simulink model "AccelCtrl_ACC_2018b"  (R2018b)
settings: Solver=FixedStepAuto  StartTime=0.0  StopTime=inf  FixedStep=0.001  RelTol=1e-3  EnableMultiTasking=on
libraries: CarMaker4SL x42, simulink x2
(part 2 of 3)

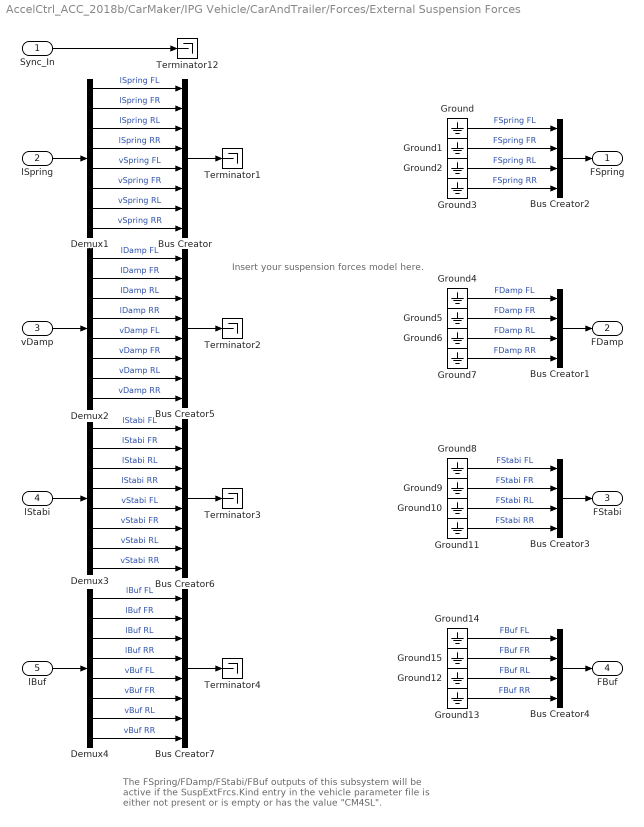
== system AccelCtrl_ACC_2018b/CarMaker/IPG Vehicle/CarAndTrailer/Forces/External Suspension Forces ==
  note: The FSpring/FDamp/FStabi/FBuf outputs of this subsystem will be
      | active if the SuspExtFrcs.Kind entry in the vehicle parameter file
      | is either not present or is empty or has the value "CM4SL".
  note: Insert your suspension forces model here.
  Sync_In : Inport
  lSpring : Inport  Port=2
  vDamp : Inport  Port=3
  lStabi : Inport  Port=4
  lBuf : Inport  Port=5
  Bus Creator{,5..7} (4 alike) : BusCreator  Inputs=8
  Bus Creator{1..4} (4 alike) : BusCreator  Inputs=4
  Demux{1..4} (4 alike) : Demux  Outputs=8
  Ground{,1..15} (16 alike) : Ground
  Terminator{1..4,12} (5 alike) : Terminator
  FSpring : Outport
  FDamp : Outport  Port=2
  FStabi : Outport  Port=3
  FBuf : Outport  Port=4
  wires:
  Bus Creator7/1 -> Terminator4/1
  Bus Creator6/1 -> Terminator3/1
  Bus Creator5/1 -> Terminator2/1
  Bus Creator/1 -> Terminator1/1
  Demux4/8 -> Bus Creator7/8  "vBuf RR"
  Demux4/7 -> Bus Creator7/7  "vBuf RL"
  Demux4/6 -> Bus Creator7/6  "vBuf FR"
  Demux4/5 -> Bus Creator7/5  "vBuf FL"
  Demux3/8 -> Bus Creator6/8  "vStabi RR"
  Demux3/7 -> Bus Creator6/7  "vStabi RL"
  Demux3/6 -> Bus Creator6/6  "vStabi FR"
  Demux3/5 -> Bus Creator6/5  "vStabi FL"
  Demux2/8 -> Bus Creator5/8  "vDamp RR"
  Demux2/7 -> Bus Creator5/7  "vDamp RL"
  Demux2/6 -> Bus Creator5/6  "vDamp FR"
  Demux2/5 -> Bus Creator5/5  "vDamp FL"
  Demux1/8 -> Bus Creator/8  "vSpring RR"
  Demux1/7 -> Bus Creator/7  "vSpring RL"
  Demux1/6 -> Bus Creator/6  "vSpring FR"
  Demux1/5 -> Bus Creator/5  "vSpring FL"
  Demux2/4 -> Bus Creator5/4  "lDamp RR"
  Demux2/3 -> Bus Creator5/3  "lDamp RL"
  Demux2/2 -> Bus Creator5/2  "lDamp FR"
  Demux2/1 -> Bus Creator5/1  "lDamp FL"
  Demux1/4 -> Bus Creator/4  "lSpring RR"
  Demux1/3 -> Bus Creator/3  "lSpring RL"
  Demux1/2 -> Bus Creator/2  "lSpring FR"
  Demux1/1 -> Bus Creator/1  "lSpring FL"
  Demux3/4 -> Bus Creator6/4  "lStabi RR"
  Demux3/3 -> Bus Creator6/3  "lStabi RL"
  Demux3/2 -> Bus Creator6/2  "lStabi FR"
  Demux3/1 -> Bus Creator6/1  "lStabi FL"
  lStabi/1 -> Demux3/1
  vDamp/1 -> Demux2/1
  lSpring/1 -> Demux1/1
  Demux4/4 -> Bus Creator7/4  "lBuf RR"
  Demux4/3 -> Bus Creator7/3  "lBuf RL"
  Demux4/2 -> Bus Creator7/2  "lBuf FR"
  Demux4/1 -> Bus Creator7/1  "lBuf FL"
  lBuf/1 -> Demux4/1
  Ground14/1 -> Bus Creator4/1  "FBuf FL"
  Ground15/1 -> Bus Creator4/2  "FBuf FR"
  Ground12/1 -> Bus Creator4/3  "FBuf RL"
  Ground13/1 -> Bus Creator4/4  "FBuf RR"
  Bus Creator4/1 -> FBuf/1
  Sync_In/1 -> Terminator12/1
  Bus Creator2/1 -> FSpring/1
  Ground/1 -> Bus Creator2/1  "FSpring FL"
  Ground1/1 -> Bus Creator2/2  "FSpring FR"
  Ground2/1 -> Bus Creator2/3  "FSpring RL"
  Ground3/1 -> Bus Creator2/4  "FSpring RR"
  Ground4/1 -> Bus Creator1/1  "FDamp FL"
  Ground5/1 -> Bus Creator1/2  "FDamp FR"
  Ground6/1 -> Bus Creator1/3  "FDamp RL"
  Ground7/1 -> Bus Creator1/4  "FDamp RR"
  Bus Creator1/1 -> FDamp/1
  Ground8/1 -> Bus Creator3/1  "FStabi FL"
  Ground9/1 -> Bus Creator3/2  "FStabi FR"
  Ground10/1 -> Bus Creator3/3  "FStabi RL"
  Ground11/1 -> Bus Creator3/4  "FStabi RR"
  Bus Creator3/1 -> FStabi/1

== system AccelCtrl_ACC_2018b/CarMaker/IPG Vehicle/CarAndTrailer/Forces/Tires ==
  note: The TireXX_Out signals will only be used if FileIdent is "CarMaker-Tire-CM4SL" in the tire parameter file!
      | An example parameter file can be found in Data/Tire/DT_CM4SL_UserTire.
  Sync_In : Inport
  TireFL_In : Inport  Port=2
  TireFR_In : Inport  Port=3
  TireRL_In : Inport  Port=4
  TireRR_In : Inport  Port=5
  Bus Creator{1..4} (4 alike) : BusCreator  Inputs=11
  Demux{1..3,8} (4 alike) : Demux  Outputs=7
  TireFL : Subsystem
  TireFR : Subsystem
  TireRL : Subsystem
  TireRR : Subsystem
  TireFL_Out : Outport
  TireFR_Out : Outport  Port=2
  TireRL_Out : Outport  Port=3
  TireRR_Out : Outport  Port=4
  wires:
  Sync_In/1 -> TireRR/1(Sync_In), TireRL/1(Sync_In), TireFR/1(Sync_In), TireFL/1(Sync_In)
  Bus Creator4/1 -> TireRR_Out/1
  Bus Creator2/1 -> TireRL_Out/1
  Bus Creator1/1 -> TireFR_Out/1
  Demux3/5 -> TireRR/6(Rim_turnv)  "Tire_In Rim_turnv"
  Demux3/4 -> TireRR/5(Rim_rotv)  "Tire_In Rim_rotv"
  Demux3/1 -> TireRR/2(Load)  "Tire_In Load"
  Demux3/7 -> TireRR/8(muRoad)  "Tire_In mu"
  Demux3/6 -> TireRR/7(InclinAngle)  "Tire_In Camber"
  Demux3/2 -> TireRR/3(vxtrans)  "Tire_In vxtrans"
  Demux3/3 -> TireRR/4(vytrans)  "Tire_In vytrans"
  TireRR/11(AlignTrq) -> Bus Creator4/11  "Tire_Out AlignTrq"
  TireRR/10(RollResist) -> Bus Creator4/10  "Tire_Out RollResist"
  TireRR/9(OverturnTrq) -> Bus Creator4/9  "Tire_Out OverturnTrq"
  TireRR/8(LoadFrc) -> Bus Creator4/8  "Tire_Out LoadFrc"
  TireRR/7(SideFrc) -> Bus Creator4/7  "Tire_Out SideFrc"
  TireRR/6(LongFrc) -> Bus Creator4/6  "Tire_Out LongFrc"
  TireRR/5(vBelt) -> Bus Creator4/5  "Tire_Out vBelt"
  TireRR/4(rBelt_eff) -> Bus Creator4/4  "Tire_Out rBelt_eff"
  TireRR/3(TurnSlp) -> Bus Creator4/3  "Tire_Out TurnSlp"
  TireRR/1(Slp) -> Bus Creator4/1  "Tire_Out Slp"
  TireRR/2(Alpha) -> Bus Creator4/2  "Tire_Out Alpha"
  Demux2/5 -> TireRL/6(Rim_turnv)  "Tire_In Rim_turnv"
  Demux2/4 -> TireRL/5(Rim_rotv)  "Tire_In Rim_rotv"
  Demux2/1 -> TireRL/2(Load)  "Tire_In Load"
  Demux2/7 -> TireRL/8(muRoad)  "Tire_In mu"
  Demux2/6 -> TireRL/7(InclinAngle)  "Tire_In Camber"
  Demux2/2 -> TireRL/3(vxtrans)  "Tire_In vxtrans"
  Demux2/3 -> TireRL/4(vytrans)  "Tire_In vytrans"
  TireRL/11(AlignTrq) -> Bus Creator2/11  "Tire_Out AlignTrq"
  TireRL/10(RollResist) -> Bus Creator2/10  "Tire_Out RollResist"
  TireRL/9(OverturnTrq) -> Bus Creator2/9  "Tire_Out OverturnTrq"
  TireRL/8(LoadFrc) -> Bus Creator2/8  "Tire_Out LoadFrc"
  TireRL/7(SideFrc) -> Bus Creator2/7  "Tire_Out SideFrc"
  TireRL/6(LongFrc) -> Bus Creator2/6  "Tire_Out LongFrc"
  TireRL/5(vBelt) -> Bus Creator2/5  "Tire_Out vBelt"
  TireRL/4(rBelt_eff) -> Bus Creator2/4  "Tire_Out rBelt_eff"
  TireRL/3(TurnSlp) -> Bus Creator2/3  "Tire_Out TurnSlp"
  TireRL/1(Slp) -> Bus Creator2/1  "Tire_Out Slp"
  TireRL/2(Alpha) -> Bus Creator2/2  "Tire_Out Alpha"
  Demux1/5 -> TireFR/6(Rim_turnv)  "Tire_In Rim_turnv"
  Demux1/4 -> TireFR/5(Rim_rotv)  "Tire_In Rim_rotv"
  Demux1/1 -> TireFR/2(Load)  "Tire_In Load"
  Demux1/7 -> TireFR/8(muRoad)  "Tire_In mu"
  Demux1/6 -> TireFR/7(InclinAngle)  "Tire_In Camber"
  Demux1/2 -> TireFR/3(vxtrans)  "Tire_In vxtrans"
  Demux1/3 -> TireFR/4(vytrans)  "Tire_In vytrans"
  TireFR/11(AlignTrq) -> Bus Creator1/11  "Tire_Out AlignTrq"
  TireFR/10(RollResist) -> Bus Creator1/10  "Tire_Out RollResist"
  TireFR/9(OverturnTrq) -> Bus Creator1/9  "Tire_Out OverturnTrq"
  TireFR/8(LoadFrc) -> Bus Creator1/8  "Tire_Out LoadFrc"
  TireFR/7(SideFrc) -> Bus Creator1/7  "Tire_Out SideFrc"
  TireFR/6(LongFrc) -> Bus Creator1/6  "Tire_Out LongFrc"
  TireFR/5(vBelt) -> Bus Creator1/5  "Tire_Out vBelt"
  TireFR/4(rBelt_eff) -> Bus Creator1/4  "Tire_Out rBelt_eff"
  TireFR/3(TurnSlp) -> Bus Creator1/3  "Tire_Out TurnSlp"
  TireFR/1(Slp) -> Bus Creator1/1  "Tire_Out Slp"
  TireFR/2(Alpha) -> Bus Creator1/2  "Tire_Out Alpha"
  Demux8/5 -> TireFL/6(Rim_turnv)  "Tire_In Rim_turnv"
  Demux8/4 -> TireFL/5(Rim_rotv)  "Tire_In Rim_rotv"
  TireFL_In/1 -> Demux8/1
  Demux8/1 -> TireFL/2(Load)  "Tire_In Load"
  Demux8/7 -> TireFL/8(muRoad)  "Tire_In mu"
  Demux8/6 -> TireFL/7(InclinAngle)  "Tire_In Camber"
  Demux8/2 -> TireFL/3(vxtrans)  "Tire_In vxtrans"
  Demux8/3 -> TireFL/4(vytrans)  "Tire_In vytrans"
  TireFL/11(AlignTrq) -> Bus Creator3/11  "Tire_Out AlignTrq"
  TireFL/10(RollResist) -> Bus Creator3/10  "Tire_Out RollResist"
  TireFL/9(OverturnTrq) -> Bus Creator3/9  "Tire_Out OverturnTrq"
  TireFL/8(LoadFrc) -> Bus Creator3/8  "Tire_Out LoadFrc"
  TireFL/7(SideFrc) -> Bus Creator3/7  "Tire_Out SideFrc"
  TireFL/6(LongFrc) -> Bus Creator3/6  "Tire_Out LongFrc"
  TireFL/5(vBelt) -> Bus Creator3/5  "Tire_Out vBelt"
  TireFL/4(rBelt_eff) -> Bus Creator3/4  "Tire_Out rBelt_eff"
  TireFL/3(TurnSlp) -> Bus Creator3/3  "Tire_Out TurnSlp"
  TireFL/1(Slp) -> Bus Creator3/1  "Tire_Out Slp"
  TireFL/2(Alpha) -> Bus Creator3/2  "Tire_Out Alpha"
  Bus Creator3/1 -> TireFL_Out/1
  TireFR_In/1 -> Demux1/1
  TireRL_In/1 -> Demux2/1
  TireRR_In/1 -> Demux3/1

== system AccelCtrl_ACC_2018b/CarMaker/IPG Vehicle/CarAndTrailer/Forces/Vehicle Forces ==
  Sync_In : Inport
  Bus Creator1 : BusCreator  Inputs=12
  Bus Creator8 : BusCreator  Inputs=16
  BusCreator1 : BusCreator  Inputs=4
  BusCreator2 : BusCreator  Inputs=9
  Demux : Demux  Outputs=16
  Demux1 : Demux  Outputs=12
  Demux2 : Demux  Outputs=13
  Forces : S-Function  FunctionName=CM_Sfun  Parameters='Forces'  SFunctionDeploymentMode=off  EnableBusSupport=off
  Terminator : Terminator
  Sync_Out : Outport
  Car.Virtual : Outport  Port=2
  Car.Aero : Outport  Port=3
  Car.Load : Outport  Port=4
  wires:
  BusCreator1/1 -> Terminator/1  "Aero IF (in)"
  Demux2/13 -> BusCreator2/9  "car Aero Trq_1 z"
  Demux2/12 -> BusCreator2/8  "car Aero Trq_1 y"
  Demux2/11 -> BusCreator2/7  "car Aero Trq_1 x"
  Demux2/10 -> BusCreator2/6  "car Aero Frc_1 z"
  Demux2/9 -> BusCreator2/5  "car Aero Frc_1 y"
  Demux2/8 -> BusCreator2/4  "car Aero Frc_1 x"
  Demux2/7 -> BusCreator2/3  "car Aero PoA_1 z"
  Demux2/6 -> BusCreator2/2  "car Aero PoA_1 y"
  Demux2/5 -> BusCreator2/1  "car Aero PoA_1 x"
  Demux2/4 -> BusCreator1/4  "car Aero tau_1"
  Demux2/3 -> BusCreator1/3  "car Aero ApproachVel_1 z"
  Demux2/2 -> BusCreator1/2  "car Aero ApproachVel_1 y"
  Demux2/1 -> BusCreator1/1  "car Aero ApproachVel_1 x"
  Demux/16 -> Bus Creator8/16  "Car Load_3 tz"
  Demux/15 -> Bus Creator8/15  "Car Load_3 ty"
  Demux/14 -> Bus Creator8/14  "Car Load_3 tx"
  Demux/13 -> Bus Creator8/13  "Car Load_3 mass"
  Demux1/12 -> Bus Creator1/12  "Car Virtual Trq_0 z"
  Demux1/11 -> Bus Creator1/11  "Car Virtual Trq_0 y"
  Demux1/10 -> Bus Creator1/10  "Car Virtual Trq_0 x"
  Demux1/9 -> Bus Creator1/9  "Car Virtual Trq_1 z"
  Demux1/8 -> Bus Creator1/8  "Car Virtual Trq_1 y"
  Demux1/7 -> Bus Creator1/7  "Car Virtual Trq_1 x"
  Demux1/6 -> Bus Creator1/6  "Car Virtual Frc_0 z"
  Demux1/5 -> Bus Creator1/5  "Car Virtual Frc_0 y"
  Demux1/4 -> Bus Creator1/4  "Car Virtual Frc_0 x"
  Sync_In/1 -> Forces/1
  Forces/1 -> Sync_Out/1
  BusCreator2/1 -> Car.Aero/1
  Demux1/1 -> Bus Creator1/1  "Car Virtual Frc_1 x"
  Demux1/2 -> Bus Creator1/2  "Car Virtual Frc_1 y"
  Demux1/3 -> Bus Creator1/3  "Car Virtual Frc_1 z"
  Forces/3 -> Demux2/1
  Forces/2 -> Demux1/1
  Bus Creator1/1 -> Car.Virtual/1
  Bus Creator8/1 -> Car.Load/1
  Demux/1 -> Bus Creator8/1  "Car Load_0 mass"
  Demux/2 -> Bus Creator8/2  "Car Load_0 tx"
  Demux/3 -> Bus Creator8/3  "Car Load_0 ty"
  Demux/4 -> Bus Creator8/4  "Car Load_0 tz"
  Demux/5 -> Bus Creator8/5  "Car Load_1 mass"
  Demux/6 -> Bus Creator8/6  "Car Load_1 tx"
  Demux/7 -> Bus Creator8/7  "Car Load_1 ty"
  Demux/8 -> Bus Creator8/8  "Car Load_1 tz"
  Demux/9 -> Bus Creator8/9  "Car Load_2 mass"
  Demux/10 -> Bus Creator8/10  "Car Load_2 tx"
  Demux/11 -> Bus Creator8/11  "Car Load_2 ty"
  Demux/12 -> Bus Creator8/12  "Car Load_2 tz"
  Forces/4 -> Demux/1

== system AccelCtrl_ACC_2018b/CarMaker/IPG Vehicle/CarAndTrailer/Trailer/CreateBus Car.Hitch.FrcTrq ==
  In1 : Inport
  Bus Creator7 : BusCreator  Inputs=6
  Demux7 : Demux  Outputs=6
  Out1 : Outport
  wires:
  In1/1 -> Demux7/1
  Bus Creator7/1 -> Out1/1
  Demux7/6 -> Bus Creator7/6  "Car Hitch Trq2Car z"
  Demux7/5 -> Bus Creator7/5  "Car Hitch Trq2Car y"
  Demux7/4 -> Bus Creator7/4  "Car Hitch Trq2Car x"
  Demux7/3 -> Bus Creator7/3  "Car Hitch Frc2Car z"
  Demux7/2 -> Bus Creator7/2  "Car Hitch Frc2Car y"
  Demux7/1 -> Bus Creator7/1  "Car Hitch Frc2Car x"

== system AccelCtrl_ACC_2018b/CarMaker/IPG Vehicle/CarAndTrailer/Trailer/CreateBus Vhcl.Motion ==
  In1 : Inport
  BusCreator : BusCreator  Inputs=15
  Demux : Demux  Outputs=15
  Out1 : Outport
  wires:
  Demux/15 -> BusCreator/15  "Vhcl YawAcc"
  Demux/14 -> BusCreator/14  "Vhcl YawVel"
  Demux/13 -> BusCreator/13  "Vhcl Yaw"
  Demux/12 -> BusCreator/12  "Vhcl PitchAcc"
  Demux/11 -> BusCreator/11  "Vhcl PitchVel"
  Demux/10 -> BusCreator/10  "Vhcl Pitch"
  Demux/9 -> BusCreator/9  "Vhcl RollAcc"
  Demux/8 -> BusCreator/8  "Vhcl RollVel"
  Demux/7 -> BusCreator/7  "Vhcl Roll"
  Demux/6 -> BusCreator/6  "Vhcl Hitch_Pos z"
  Demux/5 -> BusCreator/5  "Vhcl Hitch_Pos y"
  Demux/4 -> BusCreator/4  "Vhcl Hitch_Pos x"
  Demux/3 -> BusCreator/3  "Vhcl sRoad"
  Demux/2 -> BusCreator/2  "Vhcl Distance"
  Demux/1 -> BusCreator/1  "Vhcl v"
  In1/1 -> Demux/1
  BusCreator/1 -> Out1/1

== system AccelCtrl_ACC_2018b/CarMaker/IPG Vehicle/CarAndTrailer/Trailer/CreateBus Vhcl.PoI ==
  In1 : Inport
  Bus Creator3 : BusCreator  Inputs=18
  Demux3 : Demux  Outputs=18
  Out1 : Outport
  wires:
  Demux3/18 -> Bus Creator3/18  "Vhcl PoI_GCS Elev"
  Demux3/17 -> Bus Creator3/17  "Vhcl PoI_GCS Lat"
  Demux3/16 -> Bus Creator3/16  "Vhcl PoI_GCS Long"
  Demux3/15 -> Bus Creator3/15  "Vhcl PoI_Acc_1 z"
  Demux3/14 -> Bus Creator3/14  "Vhcl PoI_Acc_1 y"
  Demux3/13 -> Bus Creator3/13  "Vhcl PoI_Acc_1 x"
  Demux3/12 -> Bus Creator3/12  "Vhcl PoI_Vel_1 z"
  Demux3/11 -> Bus Creator3/11  "Vhcl PoI_Vel_1 y"
  Demux3/10 -> Bus Creator3/10  "Vhcl PoI_Vel_1 x"
  Demux3/9 -> Bus Creator3/9  "Vhcl PoI_Acc z"
  Demux3/8 -> Bus Creator3/8  "Vhcl PoI_Acc y"
  Demux3/7 -> Bus Creator3/7  "Vhcl PoI_Acc x"
  Demux3/6 -> Bus Creator3/6  "Vhcl PoI_Vel z"
  Demux3/5 -> Bus Creator3/5  "Vhcl PoI_Vel y"
  Demux3/4 -> Bus Creator3/4  "Vhcl PoI_Vel x"
  Demux3/3 -> Bus Creator3/3  "Vhcl PoI_Pos z"
  Demux3/2 -> Bus Creator3/2  "Vhcl PoI_Pos y"
  In1/1 -> Demux3/1
  Bus Creator3/1 -> Out1/1
  Demux3/1 -> Bus Creator3/1  "Vhcl PoI_Pos x"

== system AccelCtrl_ACC_2018b/CarMaker/IPG Vehicle/CarAndTrailer/Trailer/CreateBus Vhcl.Steering ==
  In1 : Inport
  Bus Creator3 : BusCreator  Inputs=4
  Demux : Demux
  Out1 : Outport
  wires:
  Bus Creator3/1 -> Out1/1
  Demux/1 -> Bus Creator3/1  "Vhcl Steering Ang"
  Demux/3 -> Bus Creator3/3  "Vhcl Steering AngAcc"
  Demux/2 -> Bus Creator3/2  "Vhcl Steering AngVel"
  Demux/4 -> Bus Creator3/4  "Vhcl Steering Trq"
  In1/1 -> Demux/1

== system AccelCtrl_ACC_2018b/CarMaker/IPG Vehicle/CarAndTrailer/Trailer/CreateBus Vhcl.Wheel.FL ==
  In1 : Inport
  Bus Creator3 : BusCreator  Inputs=14
  Demux3 : Demux  Outputs=14
  Out1 : Outport
  wires:
  Demux3/14 -> Bus Creator3/14  "Vhcl Wheel FL Trq_WhlBearing"
  Demux3/13 -> Bus Creator3/13  "Vhcl Wheel FL Trq_T2W"
  Demux3/12 -> Bus Creator3/12  "Vhcl Wheel FL SideSlip"
  Demux3/11 -> Bus Creator3/11  "Vhcl Wheel FL LongSlip"
  Demux3/10 -> Bus Creator3/10  "Vhcl Wheel FL vBelt"
  Demux3/9 -> Bus Creator3/9  "Vhcl Wheel FL Fz"
  Demux3/8 -> Bus Creator3/8  "Vhcl Wheel FL Fy"
  Demux3/7 -> Bus Creator3/7  "Vhcl Wheel FL Fx"
  Demux3/6 -> Bus Creator3/6  "Vhcl Wheel FL r_zxy z"
  Demux3/5 -> Bus Creator3/5  "Vhcl Wheel FL r_zxy y"
  Demux3/4 -> Bus Creator3/4  "Vhcl Wheel FL r_zxy x"
  Demux3/3 -> Bus Creator3/3  "Vhcl Wheel FL t z"
  Demux3/2 -> Bus Creator3/2  "Vhcl Wheel FL t y"
  In1/1 -> Demux3/1
  Bus Creator3/1 -> Out1/1
  Demux3/1 -> Bus Creator3/1  "Vhcl Wheel FL t x"

== system AccelCtrl_ACC_2018b/CarMaker/IPG Vehicle/CarAndTrailer/Trailer/CreateBus Vhcl.Wheel.FR ==
  In1 : Inport
  Bus Creator3 : BusCreator  Inputs=14
  Demux3 : Demux  Outputs=14
  Out1 : Outport
  wires:
  Demux3/14 -> Bus Creator3/14  "Vhcl Wheel FR Trq_WhlBearing"
  Demux3/13 -> Bus Creator3/13  "Vhcl Wheel FR Trq_T2W"
  Demux3/12 -> Bus Creator3/12  "Vhcl Wheel FR SideSlip"
  Demux3/11 -> Bus Creator3/11  "Vhcl Wheel FR LongSlip"
  Demux3/10 -> Bus Creator3/10  "Vhcl Wheel FR vBelt"
  Demux3/9 -> Bus Creator3/9  "Vhcl Wheel FR Fz"
  Demux3/8 -> Bus Creator3/8  "Vhcl Wheel FR Fy"
  Demux3/7 -> Bus Creator3/7  "Vhcl Wheel FR Fx"
  Demux3/6 -> Bus Creator3/6  "Vhcl Wheel FR r_zxy z"
  Demux3/5 -> Bus Creator3/5  "Vhcl Wheel FR r_zxy y"
  Demux3/4 -> Bus Creator3/4  "Vhcl Wheel FR r_zxy x"
  Demux3/3 -> Bus Creator3/3  "Vhcl Wheel FR t z"
  Demux3/2 -> Bus Creator3/2  "Vhcl Wheel FR t y"
  In1/1 -> Demux3/1
  Bus Creator3/1 -> Out1/1
  Demux3/1 -> Bus Creator3/1  "Vhcl Wheel FR t x"

== system AccelCtrl_ACC_2018b/CarMaker/IPG Vehicle/CarAndTrailer/Trailer/CreateBus Vhcl.Wheel.RL ==
  In1 : Inport
  Bus Creator3 : BusCreator  Inputs=14
  Demux3 : Demux  Outputs=14
  Out1 : Outport
  wires:
  Demux3/14 -> Bus Creator3/14  "Vhcl Wheel RL Trq_WhlBearing"
  Demux3/13 -> Bus Creator3/13  "Vhcl Wheel RL Trq_T2W"
  Demux3/12 -> Bus Creator3/12  "Vhcl Wheel RL SideSlip"
  Demux3/11 -> Bus Creator3/11  "Vhcl Wheel RL LongSlip"
  Demux3/10 -> Bus Creator3/10  "Vhcl Wheel RL vBelt"
  Demux3/9 -> Bus Creator3/9  "Vhcl Wheel RL Fz"
  Demux3/8 -> Bus Creator3/8  "Vhcl Wheel RL Fy"
  Demux3/7 -> Bus Creator3/7  "Vhcl Wheel RL Fx"
  Demux3/6 -> Bus Creator3/6  "Vhcl Wheel RL r_zxy z"
  Demux3/5 -> Bus Creator3/5  "Vhcl Wheel RL r_zxy y"
  Demux3/4 -> Bus Creator3/4  "Vhcl Wheel RL r_zxy x"
  Demux3/3 -> Bus Creator3/3  "Vhcl Wheel RL t z"
  Demux3/2 -> Bus Creator3/2  "Vhcl Wheel RL t y"
  In1/1 -> Demux3/1
  Bus Creator3/1 -> Out1/1
  Demux3/1 -> Bus Creator3/1  "Vhcl Wheel RL t x"

== system AccelCtrl_ACC_2018b/CarMaker/IPG Vehicle/CarAndTrailer/Trailer/CreateBus Vhcl.Wheel.RR ==
  In1 : Inport
  Bus Creator3 : BusCreator  Inputs=14
  Demux3 : Demux  Outputs=14
  Out1 : Outport
  wires:
  Demux3/14 -> Bus Creator3/14  "Vhcl Wheel RR Trq_WhlBearing"
  Demux3/13 -> Bus Creator3/13  "Vhcl Wheel RR Trq_T2W"
  Demux3/12 -> Bus Creator3/12  "Vhcl Wheel RR SideSlip"
  Demux3/11 -> Bus Creator3/11  "Vhcl Wheel RR LongSlip"
  Demux3/10 -> Bus Creator3/10  "Vhcl Wheel RR vBelt"
  Demux3/9 -> Bus Creator3/9  "Vhcl Wheel RR Fz"
  Demux3/8 -> Bus Creator3/8  "Vhcl Wheel RR Fy"
  Demux3/7 -> Bus Creator3/7  "Vhcl Wheel RR Fx"
  Demux3/6 -> Bus Creator3/6  "Vhcl Wheel RR r_zxy z"
  Demux3/5 -> Bus Creator3/5  "Vhcl Wheel RR r_zxy y"
  Demux3/4 -> Bus Creator3/4  "Vhcl Wheel RR r_zxy x"
  Demux3/3 -> Bus Creator3/3  "Vhcl Wheel RR t z"
  Demux3/2 -> Bus Creator3/2  "Vhcl Wheel RR t y"
  In1/1 -> Demux3/1
  Bus Creator3/1 -> Out1/1
  Demux3/1 -> Bus Creator3/1  "Vhcl Wheel RR t x"

== system AccelCtrl_ACC_2018b/CarMaker/VehicleControl/AccelCtrl/ACC ECU/ACC Control ==
  ACC enabled : Inport
  Target Dtct : Inport  Port=2
  Target.ds : Inport  Port=3
  Target.dv : Inport  Port=4
  Desired time gap : Inport  Port=5
  Desired speed : Inport  Port=6
  Ax is NOTSET : Constant  Value=-99999
  Desired Distance Calculation with time gap : Subsystem  TreatAsAtomicUnit=on
  Distance Control Algorithm : Subsystem  TreatAsAtomicUnit=on
  Logical Operator : Logic  AllPortsSameDT=off
  Speed Control Algorithm : Subsystem  TreatAsAtomicUnit=on
  Target detected : simulink/Logic and Bit Operations/Compare To Zero  relop=>  OutDataTypeStr=uint8  ZeroCross=off
  desired Ax : Switch  Threshold=1  SaturateOnIntegerOverflow=on
  desired or NOTSET : Switch  Threshold=1  SaturateOnIntegerOverflow=on
  Desired Ax : Outport
  wires:
  Target.dv/1 -> Distance Control Algorithm/2(Target.dv[m/s]), Desired Distance Calculation with time gap/1(Target.dv)
  Target.ds/1 -> Distance Control Algorithm/1(Target.ds[m])
  Target Dtct/1 -> Target detected/1
  Distance Control Algorithm/1("  limited ax") -> desired Ax/1
  Target detected/1 -> desired Ax/2, Logical Operator/2
  Desired Distance Calculation with time gap/1(desired distance) -> Distance Control Algorithm/3(desired distance[m])
  Desired time gap/1 -> Desired Distance Calculation with time gap/2(desired time gap)
  Desired speed/1 -> Speed Control Algorithm/1(desire speed[m/s])
  Speed Control Algorithm/1(ax speed control) -> desired Ax/3, Distance Control Algorithm/4(ax speed control)
  ACC enabled/1 -> Logical Operator/1, desired or NOTSET/2
  Logical Operator/1 -> Desired Distance Calculation with time gap/Enable
  desired or NOTSET/1 -> Desired Ax/1
  desired Ax/1 -> desired or NOTSET/1
  Ax is NOTSET/1 -> desired or NOTSET/3

== system AccelCtrl_ACC_2018b/CarMaker/VehicleControl/AccelCtrl/ACC ECU/ACC User Input ==
  ACC Active ACC/Actual Speed : Switch  Threshold=1  SaturateOnIntegerOverflow=on
  Constant : Constant
  Init Desired time gap quantity : Subsystem  TreatAsAtomicUnit=on
  Is ACC enabled : CarMaker4SL/Read CM Dict  xname=AccelCtrl.ACC.IsActive  xsync=off
  Memory : Memory
  Read Car.v[m/s] : CarMaker4SL/Read CM Dict  xname=Car.v  xsync=off
  Read Init Velocity : CarMaker4SL/Read CM Parameter  xfile=Testrun  xkey=DrivMan.Init.Velocity  xnout=1  xdefaults=0  xmuxed=on
      settings: SourceProductName=CarMaker4SL
  Read Simulation Time : CarMaker4SL/Read CM Dict  xname=Time  xsync=off
  Read User desired speed : CarMaker4SL/Read CM Dict  xname=AccelCtrl.ACC.DesiredSpd  xsync=off
  Read User desired time gap : CarMaker4SL/Read CM Dict  xname=AccelCtrl.ACC.DesiredTGap  xsync=off
  Read init desired time gap from Inf : CarMaker4SL/Read CM Parameter  xfile=Vehicle  xkey=AccelCtrl.ACC.DesrTGap  xnout=1  xdefaults=1.8  xmuxed=off
      settings: SourceProductName=CarMaker4SL
  Switch : Switch  Criteria=u2 > Threshold
  Write desired speed : CarMaker4SL/Write CM Dict  xname=AccelCtrl.ACC.DesiredSpd  xsync=off
  kmh2ms : Gain  Gain=0.28
  ACC enabled : Outport
  Desired time gap[s] : Outport  Port=2
  Desired speed[m/s] : Outport  Port=3
  wires:
  Is ACC enabled/1 -> ACC enabled/1, ACC Active ACC/Actual Speed/2
  Read Car.v[m/s]/1 -> ACC Active ACC/Actual Speed/3
  ACC Active ACC/Actual Speed/1 -> Desired speed[m/s]/1, Write desired speed/1
  Read User desired time gap/1 -> Desired time gap[s]/1
  Constant/1 -> Memory/1
  Memory/1 -> Init Desired time gap quantity/Trigger
  Read init desired time gap from Inf/1 -> Init Desired time gap quantity/1("Init desired time gap ")
  Read Init Velocity/1 -> kmh2ms/1
  Switch/1 -> ACC Active ACC/Actual Speed/1
  Read User desired speed/1 -> Switch/1
  Read Simulation Time/1 -> Switch/2
  kmh2ms/1 -> Switch/3

== system AccelCtrl_ACC_2018b/CarMaker/VehicleControl/AccelCtrl/AccelCtrl/PI-Controller ==
  delta_ax : Inport
  DM_Gas : Inport  Port=2
  AxCtrl On : Inport  Port=3
  Add : Sum  SaturateOnIntegerOverflow=on  OutDataTypeStr=Inherit: Same as first input
  Integrator : Subsystem
  Read init i_gain from Inf : CarMaker4SL/Read CM Parameter  xfile=Vehicle  xkey=AccelCtrl.i_gain  xnout=1  xdefaults=0.001  xmuxed=off
      settings: SourceProductName=CarMaker4SL
  Read init p_gain from Inf : CarMaker4SL/Read CM Parameter  xfile=Vehicle  xkey=AccelCtrl.p_gain  xnout=1  xdefaults=0.001  xmuxed=off
      settings: SourceProductName=CarMaker4SL
  Saturation : Saturate  UpperLimit=1  LowerLimit=-1
  i_gain : Product  SaturateOnIntegerOverflow=on  OutDataTypeStr=Inherit: Same as first input
  p_gain : Product  SaturateOnIntegerOverflow=on  OutDataTypeStr=Inherit: Same as first input
  Gas or Brake : Outport
  wires:
  Saturation/1 -> Gas or Brake/1
  Add/1 -> Saturation/1
  p_gain/1 -> Add/1
  delta_ax/1 -> p_gain/2, i_gain/1
  i_gain/1 -> Integrator/1(I-Part)
  AxCtrl On/1 -> Integrator/2(AxCtrl On)
  DM_Gas/1 -> Integrator/3(Init I-part)
  Integrator/1("I-part tot ") -> Add/2
  Read init p_gain from Inf/1 -> p_gain/1
  Read init i_gain from Inf/1 -> i_gain/2

== system AccelCtrl_ACC_2018b/CarMaker/VehicleControl/AccelCtrl/AccelCtrl/controlled process variable  ==
  desired ax : Inport
  Read Car.ax : CarMaker4SL/Read CM Dict  xname=Car.ax  xsync=off
  Subtract : Sum  Inputs=+-  SaturateOnIntegerOverflow=on
  delta ax : Outport
  wires:
  desired ax/1 -> Subtract/1
  Read Car.ax/1 -> Subtract/2
  Subtract/1 -> delta ax/1

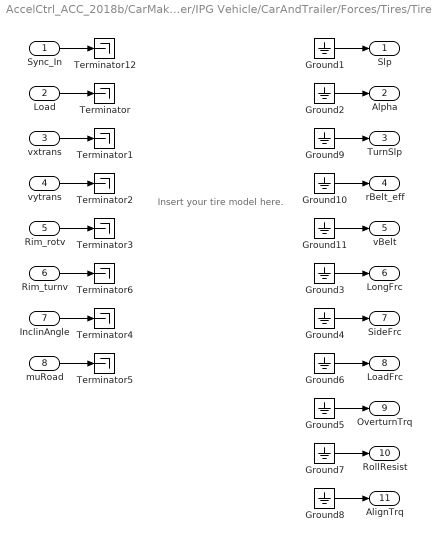
== system AccelCtrl_ACC_2018b/CarMaker/IPG Vehicle/CarAndTrailer/Forces/Tires/TireFL ==
  note: Insert your tire model here.
  Sync_In : Inport
  Load : Inport  Port=2
  vxtrans : Inport  Port=3
  vytrans : Inport  Port=4
  Rim_rotv : Inport  Port=5
  Rim_turnv : Inport  Port=6
  InclinAngle : Inport  Port=7
  muRoad : Inport  Port=8
  Ground{1..11} (11 alike) : Ground
  Terminator{,1..6,12} (8 alike) : Terminator
  Slp : Outport
  Alpha : Outport  Port=2
  TurnSlp : Outport  Port=3
  rBelt_eff : Outport  Port=4
  vBelt : Outport  Port=5
  LongFrc : Outport  Port=6
  SideFrc : Outport  Port=7
  LoadFrc : Outport  Port=8
  OverturnTrq : Outport  Port=9
  RollResist : Outport  Port=10
  AlignTrq : Outport  Port=11
  wires:
  Ground11/1 -> vBelt/1
  Ground10/1 -> rBelt_eff/1
  Ground9/1 -> TurnSlp/1
  Rim_turnv/1 -> Terminator6/1
  Sync_In/1 -> Terminator12/1
  Ground2/1 -> Alpha/1
  Ground3/1 -> LongFrc/1
  Ground4/1 -> SideFrc/1
  Ground5/1 -> OverturnTrq/1
  vxtrans/1 -> Terminator1/1
  vytrans/1 -> Terminator2/1
  Rim_rotv/1 -> Terminator3/1
  InclinAngle/1 -> Terminator4/1
  muRoad/1 -> Terminator5/1
  Load/1 -> Terminator/1
  Ground1/1 -> Slp/1
  Ground6/1 -> LoadFrc/1
  Ground7/1 -> RollResist/1
  Ground8/1 -> AlignTrq/1

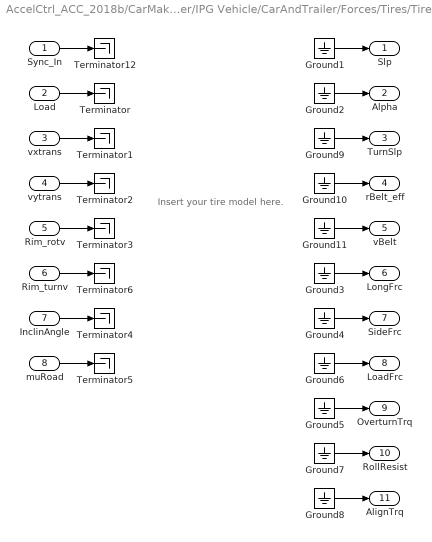
== system AccelCtrl_ACC_2018b/CarMaker/IPG Vehicle/CarAndTrailer/Forces/Tires/TireFR ==
  note: Insert your tire model here.
  Sync_In : Inport
  Load : Inport  Port=2
  vxtrans : Inport  Port=3
  vytrans : Inport  Port=4
  Rim_rotv : Inport  Port=5
  Rim_turnv : Inport  Port=6
  InclinAngle : Inport  Port=7
  muRoad : Inport  Port=8
  Ground{1..11} (11 alike) : Ground
  Terminator{,1..6,12} (8 alike) : Terminator
  Slp : Outport
  Alpha : Outport  Port=2
  TurnSlp : Outport  Port=3
  rBelt_eff : Outport  Port=4
  vBelt : Outport  Port=5
  LongFrc : Outport  Port=6
  SideFrc : Outport  Port=7
  LoadFrc : Outport  Port=8
  OverturnTrq : Outport  Port=9
  RollResist : Outport  Port=10
  AlignTrq : Outport  Port=11
  wires:
  Ground11/1 -> vBelt/1
  Ground10/1 -> rBelt_eff/1
  Ground9/1 -> TurnSlp/1
  Rim_turnv/1 -> Terminator6/1
  Sync_In/1 -> Terminator12/1
  Ground2/1 -> Alpha/1
  Ground3/1 -> LongFrc/1
  Ground4/1 -> SideFrc/1
  Ground5/1 -> OverturnTrq/1
  vxtrans/1 -> Terminator1/1
  vytrans/1 -> Terminator2/1
  Rim_rotv/1 -> Terminator3/1
  InclinAngle/1 -> Terminator4/1
  muRoad/1 -> Terminator5/1
  Load/1 -> Terminator/1
  Ground1/1 -> Slp/1
  Ground6/1 -> LoadFrc/1
  Ground7/1 -> RollResist/1
  Ground8/1 -> AlignTrq/1

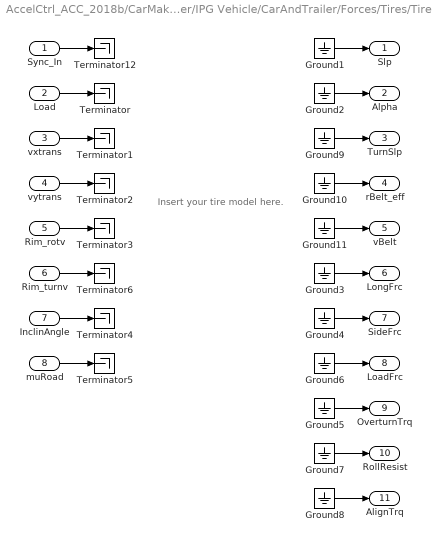
== system AccelCtrl_ACC_2018b/CarMaker/IPG Vehicle/CarAndTrailer/Forces/Tires/TireRL ==
  note: Insert your tire model here.
  Sync_In : Inport
  Load : Inport  Port=2
  vxtrans : Inport  Port=3
  vytrans : Inport  Port=4
  Rim_rotv : Inport  Port=5
  Rim_turnv : Inport  Port=6
  InclinAngle : Inport  Port=7
  muRoad : Inport  Port=8
  Ground{1..11} (11 alike) : Ground
  Terminator{,1..6,12} (8 alike) : Terminator
  Slp : Outport
  Alpha : Outport  Port=2
  TurnSlp : Outport  Port=3
  rBelt_eff : Outport  Port=4
  vBelt : Outport  Port=5
  LongFrc : Outport  Port=6
  SideFrc : Outport  Port=7
  LoadFrc : Outport  Port=8
  OverturnTrq : Outport  Port=9
  RollResist : Outport  Port=10
  AlignTrq : Outport  Port=11
  wires:
  Ground11/1 -> vBelt/1
  Ground10/1 -> rBelt_eff/1
  Ground9/1 -> TurnSlp/1
  Rim_turnv/1 -> Terminator6/1
  Sync_In/1 -> Terminator12/1
  Ground2/1 -> Alpha/1
  Ground3/1 -> LongFrc/1
  Ground4/1 -> SideFrc/1
  Ground5/1 -> OverturnTrq/1
  vxtrans/1 -> Terminator1/1
  vytrans/1 -> Terminator2/1
  Rim_rotv/1 -> Terminator3/1
  InclinAngle/1 -> Terminator4/1
  muRoad/1 -> Terminator5/1
  Load/1 -> Terminator/1
  Ground1/1 -> Slp/1
  Ground6/1 -> LoadFrc/1
  Ground7/1 -> RollResist/1
  Ground8/1 -> AlignTrq/1

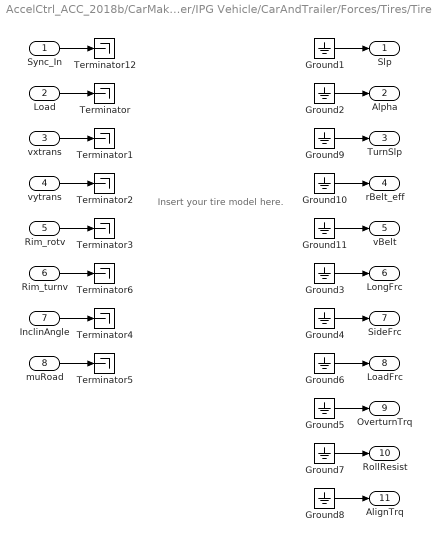
== system AccelCtrl_ACC_2018b/CarMaker/IPG Vehicle/CarAndTrailer/Forces/Tires/TireRR ==
  note: Insert your tire model here.
  Sync_In : Inport
  Load : Inport  Port=2
  vxtrans : Inport  Port=3
  vytrans : Inport  Port=4
  Rim_rotv : Inport  Port=5
  Rim_turnv : Inport  Port=6
  InclinAngle : Inport  Port=7
  muRoad : Inport  Port=8
  Ground{1..11} (11 alike) : Ground
  Terminator{,1..6,12} (8 alike) : Terminator
  Slp : Outport
  Alpha : Outport  Port=2
  TurnSlp : Outport  Port=3
  rBelt_eff : Outport  Port=4
  vBelt : Outport  Port=5
  LongFrc : Outport  Port=6
  SideFrc : Outport  Port=7
  LoadFrc : Outport  Port=8
  OverturnTrq : Outport  Port=9
  RollResist : Outport  Port=10
  AlignTrq : Outport  Port=11
  wires:
  Ground11/1 -> vBelt/1
  Ground10/1 -> rBelt_eff/1
  Ground9/1 -> TurnSlp/1
  Rim_turnv/1 -> Terminator6/1
  Sync_In/1 -> Terminator12/1
  Ground2/1 -> Alpha/1
  Ground3/1 -> LongFrc/1
  Ground4/1 -> SideFrc/1
  Ground5/1 -> OverturnTrq/1
  vxtrans/1 -> Terminator1/1
  vytrans/1 -> Terminator2/1
  Rim_rotv/1 -> Terminator3/1
  InclinAngle/1 -> Terminator4/1
  muRoad/1 -> Terminator5/1
  Load/1 -> Terminator/1
  Ground1/1 -> Slp/1
  Ground6/1 -> LoadFrc/1
  Ground7/1 -> RollResist/1
  Ground8/1 -> AlignTrq/1

== system AccelCtrl_ACC_2018b/CarMaker/VehicleControl/AccelCtrl/ACC ECU/ACC Control/Desired Distance Calculation with time gap ==
  Target.dv : Inport
  desired time gap : Inport  Port=2
  Enable : EnablePort
  Add : Sum  SaturateOnIntegerOverflow=on  OutDataTypeStr=Inherit: Same as first input
  MinMax : MinMax  Function=max  Inputs=2  SaturateOnIntegerOverflow=on  InputSameDT=on
  Product : Product  SaturateOnIntegerOverflow=on  OutDataTypeStr=Inherit: Same as first input
  Read Car.v[m/s] : CarMaker4SL/Read CM Dict  xname=Car.v  xsync=off
  Read init min distance from Inf : CarMaker4SL/Read CM Parameter  xfile=Vehicle  xkey=AccelCtrl.ACC.DistMin  xnout=1  xdefaults=20  xmuxed=off
      settings: SourceProductName=CarMaker4SL
  Write desired distance : CarMaker4SL/Write CM Dict  xname=AccelCtrl.ACC.DesiredDist  xsync=off
  desired distance : Outport  InitialOutput=0
  wires:
  Read Car.v[m/s]/1 -> Add/2
  Product/1 -> MinMax/1
  Add/1 -> Product/2
  desired time gap/1 -> Product/1
  Target.dv/1 -> Add/1
  MinMax/1 -> desired distance/1, Write desired distance/1
  Read init min distance from Inf/1 -> MinMax/2

== system AccelCtrl_ACC_2018b/CarMaker/VehicleControl/AccelCtrl/ACC ECU/ACC Control/Distance Control Algorithm ==
  Target.ds[m] : Inport
  Target.dv[m/s] : Inport  Port=2
  desired distance[m] : Inport  Port=3
  ax speed control : Inport  Port=4
  -2.5<=ax<=1 : Saturate  UpperLimit=1  LowerLimit=-2.5
  desired ax : Subsystem
  "  limited ax" : Outport  InitialOutput=0
  wires:
  ax speed control/1 -> desired ax/4(ax speed control)
  desired distance[m]/1 -> desired ax/3(desired distance[m])
  Target.dv[m/s]/1 -> desired ax/2(Target.dv[m/s])
  Target.ds[m]/1 -> desired ax/1(Target.ds[m])
  -2.5<=ax<=1/1 -> "  limited ax"/1
  desired ax/1(desired ax) -> -2.5<=ax<=1/1

== system AccelCtrl_ACC_2018b/CarMaker/VehicleControl/AccelCtrl/ACC ECU/ACC Control/Speed Control Algorithm ==
  desire speed[m/s] : Inport
  -0.35<=ax<=1 : Saturate  UpperLimit=1  LowerLimit=-0.35
  desired ax : Subsystem
  ax speed control : Outport  InitialOutput=0
  wires:
  desire speed[m/s]/1 -> desired ax/1(desire speed[m/s])
  desired ax/1(desired ax) -> -0.35<=ax<=1/1
  -0.35<=ax<=1/1 -> ax speed control/1

== system AccelCtrl_ACC_2018b/CarMaker/VehicleControl/AccelCtrl/ACC ECU/ACC User Input/Init Desired time gap quantity ==
  "Init desired time gap " : Inport
  Trigger : TriggerPort  VariantControl=Variant
  Write init time gap : CarMaker4SL/Write CM Dict  xname=AccelCtrl.ACC.DesiredTGap  xsync=off
  wires:
  "Init desired time gap "/1 -> Write init time gap/1

== system AccelCtrl_ACC_2018b/CarMaker/VehicleControl/AccelCtrl/AccelCtrl/PI-Controller/Integrator ==
  I-Part : Inport
  AxCtrl On : Inport  Port=2
  Init I-part : Inport  Port=3
  Add1 : Sum  SaturateOnIntegerOverflow=on  OutDataTypeStr=Inherit: Same as first input
  Memory : Memory
  Saturation : Saturate  UpperLimit=1  LowerLimit=-1
  Switch Ax Init I-Part : Switch  Threshold=1  SaturateOnIntegerOverflow=on
  "I-part tot " : Outport
  wires:
  Saturation/1 -> Memory/1
  Switch Ax Init I-Part/1 -> Add1/2
  Add1/1 -> Saturation/1, "I-part tot "/1
  I-Part/1 -> Add1/1
  AxCtrl On/1 -> Switch Ax Init I-Part/2
  Memory/1 -> Switch Ax Init I-Part/1
  Init I-part/1 -> Switch Ax Init I-Part/3

== system AccelCtrl_ACC_2018b/CarMaker/VehicleControl/AccelCtrl/ACC ECU/ACC Control/Distance Control Algorithm/desired ax ==
  note: desired ax = (target.ds-desired.distance)/(kd)+target.dv/kv
  note: delta_ds
  Target.ds[m] : Inport
  Target.dv[m/s] : Inport  Port=2
  desired distance[m] : Inport  Port=3
  ax speed control : Inport  Port=4
  Add : Sum  SaturateOnIntegerOverflow=on  OutDataTypeStr=Inherit: Same as first input
  Divide : Product  Inputs=*/  SaturateOnIntegerOverflow=on  OutDataTypeStr=Inherit: Same as first input
  Divide1 : Product  Inputs=*/  SaturateOnIntegerOverflow=on  OutDataTypeStr=Inherit: Same as first input
  MinMax : MinMax  Inputs=2  SaturateOnIntegerOverflow=on  InputSameDT=on
  Read init distctrl.kd from Inf : CarMaker4SL/Read CM Parameter  xfile=Vehicle  xkey=AccelCtrl.ACC.DistCtrl.kd  xnout=1  xdefaults=36  xmuxed=off
      settings: SourceProductName=CarMaker4SL
  Read init distctrl.kv from Inf1 : CarMaker4SL/Read CM Parameter  xfile=Vehicle  xkey=AccelCtrl.ACC.DistCtrl.kv  xnout=1  xdefaults=2  xmuxed=off
      settings: SourceProductName=CarMaker4SL
  Subtract : Sum  Inputs=+-  SaturateOnIntegerOverflow=on  OutDataTypeStr=Inherit: Same as first input
  desired ax : Outport
  wires:
  MinMax/1 -> desired ax/1
  ax speed control/1 -> MinMax/2
  Add/1 -> MinMax/1
  Divide1/1 -> Add/2
  Divide/1 -> Add/1
  Subtract/1 -> Divide/1
  desired distance[m]/1 -> Subtract/2
  Target.ds[m]/1 -> Subtract/1
  Target.dv[m/s]/1 -> Divide1/1
  Read init distctrl.kd from Inf/1 -> Divide/2
  Read init distctrl.kv from Inf1/1 -> Divide1/2

== system AccelCtrl_ACC_2018b/CarMaker/VehicleControl/AccelCtrl/ACC ECU/ACC Control/Speed Control Algorithm/desired ax ==
  desire speed[m/s] : Inport
  Divide : Product  Inputs=*/  SaturateOnIntegerOverflow=on  OutDataTypeStr=Inherit: Same as first input
  Read Car.v[m/s] : CarMaker4SL/Read CM Dict  xname=Car.v  xsync=off
  Read init spdctrl.kv from Inf : CarMaker4SL/Read CM Parameter  xfile=Vehicle  xkey=AccelCtrl.ACC.SpdCtrl.kv  xnout=1  xdefaults=13  xmuxed=off
      settings: SourceProductName=CarMaker4SL
  Sum : Sum  Inputs=|+-  SaturateOnIntegerOverflow=on  OutDataTypeStr=Inherit: Same as first input
  desired ax : Outport
  wires:
  Divide/1 -> desired ax/1
  desire speed[m/s]/1 -> Sum/1
  Read Car.v[m/s]/1 -> Sum/2
  Sum/1 -> Divide/1
  Read init spdctrl.kv from Inf/1 -> Divide/2

== matlab function AccelCtrl_ACC_2018b/CarMaker/VehicleControl/AccelCtrl/lowerCtrl /fcn  ==
  data: cx input; cy input; len input; steering output; yaw input; y_his input; v input; x_his input size=1; current_ind output; lat output
function [steering,current_ind, lat] = fcn(cx,cy,len,yaw,y_his, v,x_his)
if len == 0
    steering = 0; 
%     x= 0;
%     y = 0;
    current_ind = 0;
lat = 0;
    return;
end
x = x_his; y = y_his;
% [x,y] = update(x_his,y_his,yaw,v);
[lat,current_ind]= calc_current_index(x,y, cx,cy);
if current_ind == length(cx)
    steering = 0;
else
    steering = -1.2 * lat ;
end
end


function [x, y] = update(x_his,y_his, yaw, v)
    dt = 0.001;
    x = x_his + v * cos(yaw) * dt;
    y = y_his + v * sin(yaw) * dt;
%     yaw = yaw + v / L * tan(delta) * dt;
%     v = v + a * dt;
end

function [lat,current_ind]= calc_current_index(x,y, cx,cy)
N =  length(cx);
Distance = zeros(N,1);
for i = 1:N
    Distance(i) =  sqrt((cx(i)-x)^2 + (cy(i)-y)^2);
end
[value, location]= min(Distance);
current_ind = location;
lat = value;
if cy(current_ind)>y
        lat = - lat; 
else
        lat = lat;
end
end

== matlab function AccelCtrl_ACC_2018b/CarMaker/VehicleControl/AccelCtrl/Subsystem1/module_smooth  ==
  data: a0 input; cx output size=1000; a1 input; a2 input; a3 input; b0 input; b1 input; b2 input; b3 input; velocity input; indicator input; Flag input; P_alpha input; P_beta input; P_lateral_offset input; P_MAX_ITER input; P_TOL input; P_MAX_KAPPA input; cy output size=1000; LENGTH output; x_off input
function [cx,cy,LENGTH]= LineGeneration(a0,a1,a2,a3, b0,b1,b2,b3,velocity,indicator,Flag,P_alpha,P_beta,P_lateral_offset,...
    P_MAX_ITER,P_TOL, P_MAX_KAPPA,x_off)
%% the main function, which is used to generate changing lane curve dynamically    
    if Flag ~= 1
        cx = [];
        cy = [];
        LENGTH = 0;
        return;
    end
       
    LEN = calculateLEN(velocity);
    reference_1 = reference_line_generator(a0,a1,a2,a3, b0,b1,b2,b3,LEN);
    S = 0;
    D0 = 0.5 * (a0 + b0);
    Ti = LEN;
    Di = abs(P_lateral_offset) * indicator;% indicator signal should be positive when turning left, and vice versa.
    [ref_bezier] = ref_bezier_generation(reference_1, D0,Ti,Di);
    trajs_new_origin = reference_generation(reference_1, ref_bezier);
    trajs_new = PathSmoothing(trajs_new_origin, P_alpha, P_beta,P_MAX_ITER,P_TOL, P_MAX_KAPPA);
    delta_heading_rad = calculat_delta_heading(reference_1, trajs_new);
    delta_heading_deg = rad_to_deg(delta_heading_rad);
    kappa = calculate_kappa(trajs_new);
    output = [trajs_new,delta_heading_rad,kappa];
    cx = output(:,1)+ x_off;
    cy = output(:,2);
    LENGTH = length(cx);
end

function LEN = calculateLEN(velocity)
    LEN = velocity * 3.6 + 30;
    LEN = round(LEN);
    
    if LEN == 0
        fprintf('LEN calculation error. \r')
    end
end

function [ref_bezier] = ref_bezier_generation(reference_1, D0, Ti, Di)
%% this function generate bezier curve information 
% input: the centerline reference_1, bezier curve control points
% output: the matrix is in dimension of n by 2, with its first col
% longitudinal integration length, second col lateral offset with respect
% to center line.
% notice: shifting to left is positive, and vice versa. 
S = 0;
    ref_bezier = [[],[]];
    index =1;
    while S < Ti
        p = Bezierfrenet_5(D0, Ti, Di,S);
        ref_bezier =[ref_bezier; p];
        S = S + sqrt((reference_1(index+1,1)-reference_1(index,1))^2 + ...
            (reference_1(index+1,2)-reference_1(index,2))^2);
        index = index + 1;
    end
end

function [delta_heading] = calculat_delta_heading(center_line, traj_new)
    LEN = min(length(center_line), length(traj_new));
    delta_heading = [0];
    for i = 1: LEN-1
        x1 = center_line(i+1,1) - center_line(i,1);
        y1 = center_line(i+1,2) - center_line(i,2);
        x2 = traj_new(i+1,1) - traj_new(i,1);
        y2 = traj_new(i+1,2) - traj_new(i,2);
        delta_theta =  (x1 * x2 + y1 * y2) / (sqrt(x1^2 + y1^2) * sqrt(x2^2 + y2^2));
        delta_heading =  [delta_heading; acos(delta_theta)];
    end
end

function [reference] = reference_line_generator(a0,a1,a2,a3, b0,b1,b2,b3, LEN)
%% in this function, we use the left and right lane polynomials to generate
% a reference center line
% input: left lane polynomials, right lane polynomials, LEN(length of reference)
% output: reference center line polynomials
reference = [[],[]];
if LEN == 0
    fprintf('LEN = 0, reference cannot be generated. \r')
    return;
end

for i = 0:0.2:LEN
    y = 0.5 * ( (a0 + a1 * i + a2 * i^2 + a3 * i^3) + (b0 + b1 * i + b2 * i^2 + b3 * i^3));
    reference =  [reference; [i,y]];
end
end

function y = f_a(a0, a1, a2, a3, x)
%% calculate polynomial y values
    y = a0 + a1 * x + a2 * x^2 + a3 * x^3;
end

function y = f_b(b0, b1, b2, b3, x)
%% calculate polynomial y values
    y = b0 + b1 * x + b2 * x^2 + b3 * x^3;
end

function y = deg_to_rad(x)
%% deg to rad unit switch
    y = x * pi / 180;
end

function y = rad_to_deg(x)
%% rad to degree unit switch
    y = x * 180 / pi;
end

function [reference] = reference_line_generator_frenet(a0,a1,a2,a3, b0,b1,b2,b3, LEN)
%% this function generates center line in discrete form
% input: the left lane and right lane polynomials parameters, and
% longitudinal LEN(how long we want to generate such a curve)
% output: using frenet method to generate the ceterline position in x and
% y

if LEN == 0
    fprintf('LEN = 0, reference cannot be generated. \r');
    return;
end

S = 0;
iter = 0;
x_a = 0;
x_b = 0;

delta_x = 0.02;
RESOLUTION = 0.2;
y_a_pre = f_a(a0,a1,a2,a3, x_a);
y_b_pre = f_b(b0,b1,b2,b3, x_b);
reference = [x_a, 0.5*(y_a_pre + y_b_pre)];
while S < LEN

    s_a = 0;
    s_b = 0;
    while s_a < RESOLUTION
        x_a = x_a + delta_x;
        y_a = f_a(a0,a1,a2,a3, x_a);
        s_a = s_a + sqrt( delta_x^2 + (y_a - y_a_pre)^2);
        y_a_pre = y_a;
    end
    
    while s_b < RESOLUTION 
        x_b = x_b + delta_x;
        y_b = f_b(b0,b1,b2,b3, x_b);
        s_b = s_b + sqrt( delta_x^2 + (y_b - y_b_pre)^2);
        y_b_pre = y_b;
    end
    
    S = S + RESOLUTION;
    reference = [reference; [0.5*(x_a + x_b), 0.5*(y_a + y_b) ]];
    
    iter = iter + 1;
    if iter >= 5000
        print("while loop too long, missing error! \r")
        break;
    end
    
end
end

function [p] = Bezierfrenet_5(D0, Ti, Di,t)
%% this function provides the bezier curve information. 
% when given control points information, it can generate y values based on
% given x values.
    p0 = [ 0, D0];
    p1 = [0.25 * Ti, D0];
    p2= [0.5 *Ti, D0];
    p3 =[ 0.5 * Ti, Di];
    p4 =[ 0.75 * Ti, Di];
    p5 = [Ti, Di];
  %generate a fifth order bezier curve

    p= (1-(t)/Ti)^5*p0 + 5*(1-(t)/Ti)^4*((t)/Ti)*p1 + 10*(1-(t)/Ti)^3*((t)/Ti)^2*p2 +...
     10*(1-(t)/Ti)^2*((t)/Ti)^3*p3 +5*(1-(t)/Ti)*((t)/Ti)^4*p4 + ((t)/Ti)^5*p5;

end
 
function [trajs_new] = reference_generation(trajs_local, p_store)
%% this function provides method of generating changing lane discrete positions.    
% inputs: here the trajs_local is a vector<vector<double>>,with its dimension
%n by 2, the p_store store the information Bezier curve generaion
%function creates, which are longitudinal 's' and 'lateral offset', which
%is also in dimension of n by 2. 
%output: with the two inputs info, we are able to generate under vehicle
%coordinate the changing lane positions by doing position shift, based on
%the original trajs_local, in frenet direction with offset info provided by
%p_store.
if (isempty(trajs_local)) || (length(trajs_local) == 0)
    fprintf('reference trajs is not well generated! \r');
    trajs_new= [];
    return;
end

if isempty(p_store) || (length(p_store) == 0)
    fprintf('offset Bezier curve is not well generated! \r');
    trajs_new= [];
    return;
end

    trajs_new = [[ ],[ ]];
    for i = 1: min(length(p_store), length(trajs_local))
%         if (i + current_index) > length(waypoint)
%             break;
%         end
        d = p_store(i,2);
        if trajs_local(i,1) == 0
            theta = 0;
        else
            theta = atan(trajs_local(i,2) / trajs_local(i,1));
        end
        
        if (theta>-pi/2 && theta <=0)
            x = trajs_local(i,1) - d * sin(theta);
            y = trajs_local(i,2) + d * cos(theta);
            trajs_new = [trajs_new ; [x,y]];
        elseif (theta>0 && theta < pi/2)
            x = trajs_local(i,1) - d * sin(theta);
            y = trajs_local(i,2) + d * cos(theta);
            trajs_new = [trajs_new ; [x,y]];    
        else
           fprintf("it seems that the reference line is unacceptable!");
        end
    end
end

function optPath = PathSmoothing(path, alpha, beta,P_MAX_ITER,P_TOL, P_MAX_KAPPA)
    optPath=path;%
    iter = 0;
    COND = 1;
    while COND == 1 
%         change=0;
        for ip=2:(length(path(:,1))-1) 
          optPath(ip,:)=optPath(ip,:)-alpha*(optPath(ip,:)-path(ip,:));
            term_dx_1 = 2*optPath(ip,:)-optPath(ip-1,:)-optPath(ip+1,:);
%             term_dx_2 = optPath(ip-2,:) - 4*optPath(ip-1,:) + 6 * optPath(ip,:)...
%                 -4 * optPath(ip+1,:) - optPath(ip+2,:);
            optPath(ip,:) = optPath(ip,:)-beta * term_dx_1;
%           change=change+norm(optPath(ip,:)-prePath);
        end
        kappa = calculate_kappa(optPath);
        
        iter = iter + 1
        
        change = zeros(1,length(optPath));
        for i = 1:length(optPath)
            change(i) = norm(optPath(i,:)-path(i,:));
            if max(abs(change)) >= P_TOL % 0.7
                COND = 2
                 [value, loc] = max(abs(change))
                break;
            end
        end
        
        if iter > P_MAX_ITER % 10000
            COND = 3;
        end
        
        sum = 0;
        for i = 1: length(kappa)    
            if abs(kappa(i)) > P_MAX_KAPPA %0.002
               sum = sum + 1; 
            end
        end
        
        if sum == 0
            COND = 4
        end
                   
    end
end


function [kappa] = calculate_kappa(trajs_new)

%% this function provide the method of generating a sequence of curvature(kappa) 
% input: a sequence of discrete points with position x and y.
% output: a sequence of kappa on each point.
% notice: vehicle turning right has negative curvature, and vice versa.

if (isempty(trajs_new)) || (length(trajs_new) == 0)
    fprintf('changing lane trajs is not well generated! \r');
    kappa = zeros(length(trajs_new),1);
    return;
end

    pd = zeros(length(trajs_new),1);
    pdd = zeros(length(trajs_new),1);
    kappa = zeros(length(trajs_new),1);
    
    % calculate the first derivatives
    
    for i = 1:length(trajs_new)-1
        
        if (trajs_new(i+1,1)-trajs_new(i,1)) == 0
            denominator_pd = 0.001;
        else
            denominator_pd = trajs_new(i+1,1)-trajs_new(i,1);
        end
        
        pd(i) = (trajs_new(i+1,2)-trajs_new(i,2))/denominator_pd;   
    end
    pd(length(trajs_new)) = pd(length(trajs_new)-1);
    % calculate the second derivatives
    pdd(1) = 0;
    for i =2: length(trajs_new)-1
        
        if (0.5*(-trajs_new(i-1,1)+trajs_new(i+1,1)))^2 == 0
            denominator_pdd = 0.001;
        else
            denominator_pdd = 0.5*(-trajs_new(i-1,1)+trajs_new(i+1,1))^2;
        end
        
        pdd(i) = (trajs_new(i+1,2)-2*trajs_new(i,2) +...
            trajs_new(i-1,2))/denominator_pdd;
    end
    pdd(length(trajs_new)) = pdd(length(trajs_new)-1);
    
    for i  = 1:length(trajs_new)
        kappa(i) = (pdd(i))/((1+pd(i)^2)^(1.5));
    end
end

function [location] = update_trajs(velocity,trajs_new,delta_t)
%% this function dynamically update trajs_new for LKA system
S = velocity * delta_t;
    s = 0;
    for i = 1: length(trajs_new)
        s = s + sqrt((trajs_new(i+1,1) - trajs_new(i,1))^2 + ...
            (trajs_new(i+1,2) - trajs_new(i,2))^2);
        if s>= S
            break;
        end
    end
end

== matlab function AccelCtrl_ACC_2018b/CarMaker/VehicleControl/AccelCtrl/MATLAB Function ==
  data: steering input; y output; lat input; error output; ind input; len input
function [y, error]= fcn(steering, lat,ind,len)
    error = abs(-1.75 - lat);
    if error < 0.4 || ind >= 300
        y = 0.7 * (-1.75 - lat);
    else
        y = steering;
    end
end
